simulink model "demod"  (Simulink 6.6)
settings: Solver=VariableStepDiscrete  SolverMode=SingleTasking  StartTime=0.0  StopTime=32768/12.8e6  RelTol=1e-3
PreLoadFcn:
  | load_downconverter_input
undefined symbols (not defined in the file): dfilt, get
libraries: xbsIndex_r4 x12, dsparch4 x3, dspsigops x2, dspsnks4 x2
settings Model: Creator=lcrockett  LastModifiedBy=lcrockett
settings DataIOCC: SignalLoggingName=sigsOut
settings OptimizationCC: InlineParams=on
settings DebuggingCC: SignalResolutionControl=TryResolveAllWithWarning  SolverPrmCheckMsg=none  MultiTaskDSMMsg=warning  MultiTaskCondExecSysMsg=none  StrictBusMsg=None
settings HardwareCC: TargetUnknown=on
settings RTWCC: IncludeERTFirstTime=on
settings GRTTargetCC: ModelReferenceCompliant=off  MatFileLogging=off

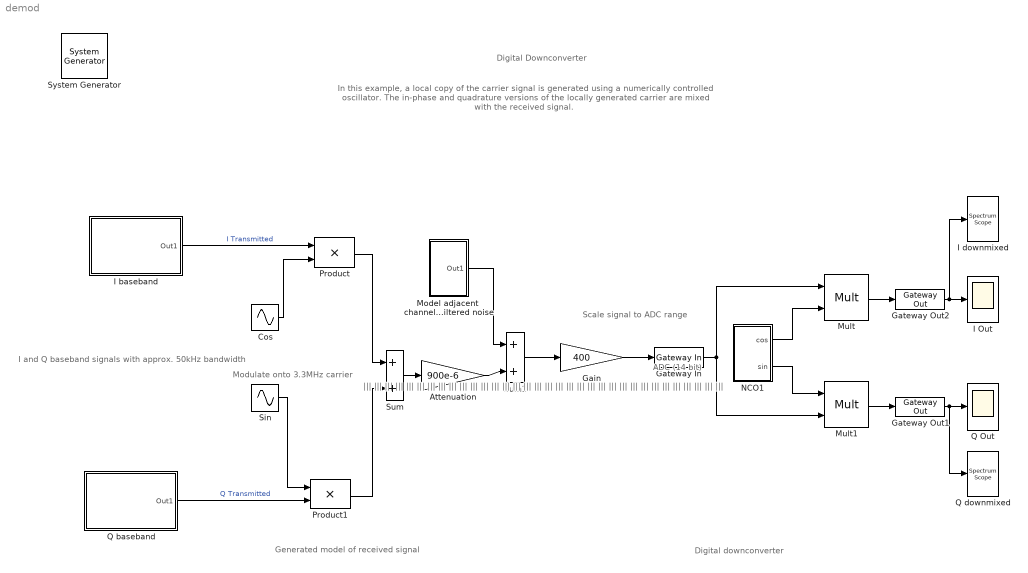
== system demod ==
  note: I and Q baseband
      | signals with approx.
      | 50kHz bandwidth
  note: Modulate onto
      | 3.3MHz carrier
  note: Digital Downconverter
  note: |||
      | |||
      | |||
      | |||
      | |||
      | |||
      | |||
      | |||
      | |||
      | |||
      | |||
      | |||
      | |||
      | |||
      | |||
      | |||
      | |||
      | |||
      | |||
      | |||
      | |||
      | |||
      | |||
      | |||
      | |||
      | |||
      | |||
      | |||
      | |||
      | |||
      | |||
      | |||
      | |||
      | |||
  note: Generated model of received signal
  note: Digital downconverter
  note: Scale signal
      | to ADC range
  note: ADC (14 bit)
  note: In this example, a local copy of the carrier signal is generated using a numerically controlled oscillator.
      | The in-phase and quadrature versions of the locally generated carrier are mixed with the received signal.
  " System Generator" : xbsIndex_r4/ System Generator  Tag=genX  SystemSampleTime=-1  xilinxfamily=virtex2p  part=xc2vp30  speed=-7  package=ff896  synthesis_tool=XST  clock_wrapper=Clock Enables  directory=./netlist_03  testbench=off  simulink_period=1/12.8e6  sysclk_period=78.125  dcm_input_clock_period=100  incr_netlist=off  trim_vbits=Everywhere in SubSystem  dbl_ovrd=According to Block Masks  core_generation=According to Block Masks  run_coregen=off  deprecated_control=off  eval_field=0  block_type=sysgen
      settings: block_version=9.2.01
  Attenuation : Gain  Gain=900e-6  SaturateOnIntegerOverflow=on
  Cos : Sin  Frequency=2*pi*3.30999970436096e6  Phase=pi/2  SampleTime=1/12.8e6
  Gain : Gain  Gain=400  SaturateOnIntegerOverflow=on
  Gateway In : xbsIndex_r4/Gateway In  arith_type="Signed  (2's comp)"  n_bits=14  bin_pt=13  quantization="Round  (unbiased: +/- Inf)"  overflow=Saturate  period=1/12.8e6  dbl_ovrd=off  timing_constraint=None  locs_specified=off  LOCs={}  block_type=gatewayin
      settings: infoedit="Gateway in block.  Converts inputs of type Simulink integer, double and fixed point to  Xilinx fixed point type.<P><P>Hardware notes:  In hardware these blocks become top level input ports."  xl_area=[0, 0, 0, 0, 0, 0, 0]  block_version=VER_STRING_GOES_HERE
  Gateway Out1 : xbsIndex_r4/Gateway Out  hdl_port=on  timing_constraint=None  locs_specified=off  LOCs={}  block_type=gatewayout
      settings: infoedit="Gateway out block.  Converts Xilinx fixed point inputs into ouputs of type Simulink integer, double, or fixed point.<P><P>Hardware notes:  In hardware these blocks become top level output ports or are discarded, depending on how they are configured."  xl_area=[0, 0, 0, 0, 0, 0, 0]  block_version=VER_STRING_GOES_HERE
  Gateway Out2 : xbsIndex_r4/Gateway Out  hdl_port=on  timing_constraint=None  locs_specified=off  LOCs={}  block_type=gatewayout
      settings: infoedit="Gateway out block.  Converts Xilinx fixed point inputs into ouputs of type Simulink integer, double, or fixed point.<P><P>Hardware notes:  In hardware these blocks become top level output ports or are discarded, depending on how they are configured."  xl_area=[0, 0, 0, 0, 0, 0, 0]  block_version=VER_STRING_GOES_HERE
  I Out : Scope
      settings: TimeRange=0.003  YMin=-1  YMax=1  DataFormat=Structure  MaxDataPoints=32768
  I baseband : Subsystem
  I downmixed : dspsnks4/Spectrum Scope  DialogController=dspdialog.SpectrumScope  DialogControllerArgs=DataTag2  SystemSampleTime=-1  ScopeProperties=on  Domain=Frequency  HorizSpan=1  UseBuffer=on  BufferSize=128  Overlap=64  inpFftLenInherit=on  FFTlength=1024  numAvg=5  DisplayProperties=off  AxisGrid=on  Memory=off  FrameNumber=on  AxisLegend=off  AxisZoom=off  OpenScopeAtSimStart=on  OpenScopeImmediately=off  FigPos=get(0,'defaultfigureposition')  AxisProperties=off  XUnits=Hertz  XRange=[0...Fs/2]  InheritXIncr=on  XIncr=1.0  XLabel=Samples  XLimit=Auto  YUnits=dB  XMax=1  XMin=0  YLabel=Magnitude, dB  LineProperties=off  wintypeSpecScope=Hann  RsSpecScope=50  betaSpecScope=5  winsampSpecScope=Periodic
      settings: YMin=-30  YMax=0
  Model adjacent  channels with  filtered noise : Subsystem
  Mult : xbsIndex_r4/Mult  precision=User Defined  arith_type="Signed  (2's comp)"  n_bits=15  bin_pt=14  quantization=Truncate  overflow=Wrap  en=off  latency=3  dbl_ovrd=off  use_behavioral_HDL=off  use_embedded=on  opt=Speed  optimum_pipeline=off  pipeline=on  use_rpm=on  placement_style=Rectangular shape  block_type=mult
      settings: infoedit=Hardware notes: To use the internal pipeline stage of the dedicated multiplier you must select 'Pipeline for maximum performance'.  xl_area=[0, 0, 0, 0, 0, 0, 0]  block_version=VER_STRING_GOES_HERE
  Mult1 : xbsIndex_r4/Mult  precision=User Defined  arith_type="Signed  (2's comp)"  n_bits=15  bin_pt=14  quantization=Truncate  overflow=Wrap  en=off  latency=3  dbl_ovrd=off  use_behavioral_HDL=off  use_embedded=on  opt=Speed  optimum_pipeline=off  pipeline=on  use_rpm=on  placement_style=Rectangular shape  block_type=mult
      settings: infoedit=Hardware notes: To use the internal pipeline stage of the dedicated multiplier you must select 'Pipeline for maximum performance'.  xl_area=[0, 0, 0, 0, 0, 0, 0]  block_version=VER_STRING_GOES_HERE
  NCO1 : Subsystem
  Product : Product  SaturateOnIntegerOverflow=on
  Product1 : Product  SaturateOnIntegerOverflow=on
  Q Out : Scope
      settings: TimeRange=0.003  YMin=-1  YMax=1  DataFormat=Structure  MaxDataPoints=32768
  Q baseband : Subsystem
  Q downmixed : dspsnks4/Spectrum Scope  DialogController=dspdialog.SpectrumScope  DialogControllerArgs=DataTag5  SystemSampleTime=-1  ScopeProperties=on  Domain=Frequency  HorizSpan=1  UseBuffer=on  BufferSize=128  Overlap=64  inpFftLenInherit=on  FFTlength=1024  numAvg=5  DisplayProperties=off  AxisGrid=on  Memory=off  FrameNumber=on  AxisLegend=off  AxisZoom=off  OpenScopeAtSimStart=on  OpenScopeImmediately=off  FigPos=get(0,'defaultfigureposition')  AxisProperties=off  XUnits=Hertz  XRange=[0...Fs/2]  InheritXIncr=on  XIncr=1.0  XLabel=Samples  XLimit=Auto  YUnits=dB  XMax=1  XMin=0  YLabel=Magnitude, dB  LineProperties=off  wintypeSpecScope=Hann  RsSpecScope=50  betaSpecScope=5  winsampSpecScope=Periodic
      settings: YMin=-30  YMax=0
  Sin : Sin  Frequency=2*pi*3.30999970436096e6  SampleTime=1/12.8e6
  Sum : Sum  Inputs=|++  SaturateOnIntegerOverflow=on
  Sum1 : Sum  Inputs=|++  SaturateOnIntegerOverflow=on
  wires:
  I baseband/1(Out1) -> Product/1  "I Transmitted"
  Q baseband/1(Out1) -> Product1/2  "Q Transmitted"
  Product/1 -> Sum/1
  Product1/1 -> Sum/2
  Sum/1 -> Attenuation/1
  Attenuation/1 -> Sum1/2
  Model adjacent  channels with  filtered noise/1(Out1) -> Sum1/1
  Sum1/1 -> Gain/1
  Gain/1 -> Gateway In/1
  Gateway In/1 -> Mult/1, Mult1/2
  Gateway Out2/1 -> I Out/1, I downmixed/1
  Gateway Out1/1 -> Q Out/1, Q downmixed/1
  Mult1/1 -> Gateway Out1/1
  Mult/1 -> Gateway Out2/1
  NCO1/2(sin) -> Mult1/1
  NCO1/1(cos) -> Mult/2
  Sin/1 -> Product1/1
  Cos/1 -> Product/2

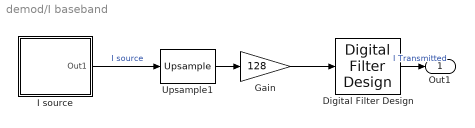
== system demod/I baseband ==
  Digital Filter Design : dsparch4/Digital Filter Design  SystemSampleTime=-1  mwdsp_browser_bugfix_var=off
  Gain : Gain  Gain=128
  I source : Subsystem
  Upsample1 : dspsigops/Upsample  N=128  phase=0  ic=0  mode=Maintain input frame size
  Out1 : Outport
  wires:
  I source/1(Out1) -> Upsample1/1  "I source"
  Upsample1/1 -> Gain/1
  Gain/1 -> Digital Filter Design/1
  Digital Filter Design/1 -> Out1/1  "I Transmitted"

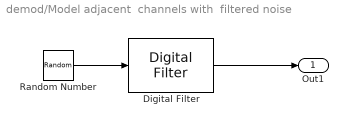
== system demod/Model adjacent  channels with  filtered noise ==
  Digital Filter : dsparch4/Digital Filter  DialogController=dspdialog.DigitalFilter  DialogControllerArgs=DataTag3  TypePopup=FIR (all zeros)  IIRFiltStruct=Direct form II transposed  AllPoleFiltStruct=Direct form  FIRFiltStruct=Direct form  CoeffSource=Specify via dialog  NumCoeffs=BandStop  DenCoeffs=[1]  BiQuadCoeffs=[1 0.3 0.4 1 0.1 0.2]  LatticeCoeffs=[0.2 0.4]  denIgnore=on  FiltPerSampPopup=One filter per frame  IC=0  ICnum=0  ICden=0  roundingMode=Floor  overflowMode=off  ScaleValues=1  scaleValueFracLength=14  stageInFracLength=15  stageOutFracLength=15  FilterSource=Specify via dialog  dfiltObjectName=dfilt.dffir([1 2 1])
  Random Number : RandomNumber  Variance=3.4e-7  Seed=1  SampleTime=1/12.8e6
  Out1 : Outport
  wires:
  Random Number/1 -> Digital Filter/1
  Digital Filter/1 -> Out1/1

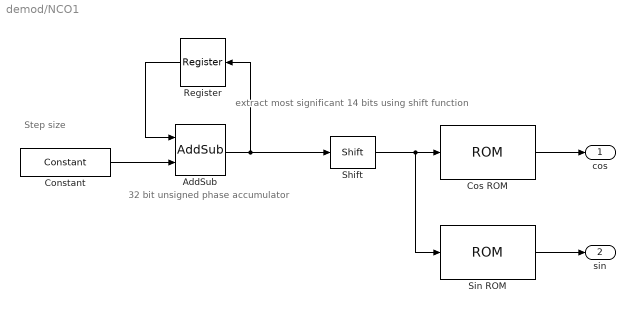
== system demod/NCO1 ==
  note: extract most
      | significant
      | 14 bits using
      | shift function
  note: 32 bit unsigned phase accumulator
  note: Step size
  AddSub : xbsIndex_r4/AddSub  mode=Addition  use_carryin=off  use_carryout=off  en=off  latency=0  precision=User Defined  arith_type=Unsigned  n_bits=32  bin_pt=0  quantization=Truncate  overflow=Wrap  dbl_ovrd=off  use_behavioral_HDL=on  pipelined=off  use_rpm=on  block_type=addsub
      settings: xl_area=[0, 0, 0, 0, 0, 0, 0]  block_version=VER_STRING_GOES_HERE
  Constant : xbsIndex_r4/Constant  arith_type=Unsigned  const=1.11065e9  n_bits=32  bin_pt=0  explicit_period=on  period=1/12.8e6  equ=P=C  opselect=C  inp2=PCIN>>17  opr=+  inp1=P  carry=CIN  dbl_ovrd=off  block_type=constant
      settings: block_version=VER_STRING_GOES_HERE
  Cos ROM : xbsIndex_r4/ROM  depth=16384  initVector=cos(pi*(0:16383)/8192)  distributed_mem=Block RAM  rst=off  init_reg=0  en=off  latency=1  arith_type="Signed  (2's comp)"  n_bits=14  bin_pt=13  dbl_ovrd=off  optimize=Area  use_rpm=off  block_type=sprom
      settings: xl_area=[0, 0, 0, 0, 0, 0, 0]  block_version=VER_STRING_GOES_HERE
  Register : xbsIndex_r4/Register  Orientation=left  init=0  rst=off  en=off  dbl_ovrd=off  block_type=register
      settings: xl_area=[0, 0, 0, 0, 0, 0, 0]  block_version=VER_STRING_GOES_HERE
  Shift : xbsIndex_r4/Shift  shift_dir=Right  shift_bits=18  en=off  latency=0  precision=User Defined  arith_type=Unsigned  n_bits=14  bin_pt=0  quantization=Truncate  overflow=Wrap  dbl_ovrd=off  block_type=shift
      settings: xl_area=[0, 0, 0, 0, 0, 0, 0]  block_version=VER_STRING_GOES_HERE
  Sin ROM : xbsIndex_r4/ROM  depth=16384  initVector=sin(pi*(0:16383)/8192)  distributed_mem=Block RAM  rst=off  init_reg=0  en=off  latency=1  arith_type="Signed  (2's comp)"  n_bits=14  bin_pt=13  dbl_ovrd=off  optimize=Area  use_rpm=off  block_type=sprom
      settings: xl_area=[0, 0, 0, 0, 0, 0, 0]  block_version=VER_STRING_GOES_HERE
  cos : Outport
  sin : Outport  Port=2
  wires:
  Constant/1 -> AddSub/2
  AddSub/1 -> Register/1, Shift/1
  Register/1 -> AddSub/1
  Sin ROM/1 -> sin/1
  Cos ROM/1 -> cos/1
  Shift/1 -> Cos ROM/1, Sin ROM/1

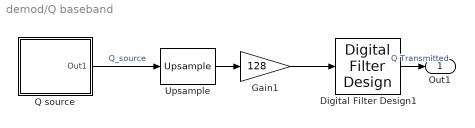
== system demod/Q baseband ==
  Digital Filter Design1 : dsparch4/Digital Filter Design  SystemSampleTime=-1  mwdsp_browser_bugfix_var=off
  Gain1 : Gain  Gain=128
  Q source : Subsystem
  Upsample : dspsigops/Upsample  N=128  phase=0  ic=0  mode=Maintain input frame size
  Out1 : Outport
  wires:
  Q source/1(Out1) -> Upsample/1  "Q_source"
  Upsample/1 -> Gain1/1
  Gain1/1 -> Digital Filter Design1/1
  Digital Filter Design1/1 -> Out1/1  "Q Transmitted"

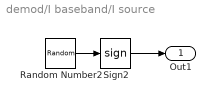
== system demod/I baseband/I source ==
  Random Number2 : RandomNumber  Seed=777  SampleTime=1/100e3
  Sign2 : Signum
  Out1 : Outport
  wires:
  Random Number2/1 -> Sign2/1
  Sign2/1 -> Out1/1

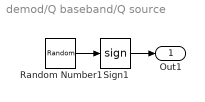
== system demod/Q baseband/Q source ==
  Random Number1 : RandomNumber  Seed=99  SampleTime=1/100e3
  Sign1 : Signum
  Out1 : Outport
  wires:
  Random Number1/1 -> Sign1/1
  Sign1/1 -> Out1/1
